simulink model "nonlinear_model"  (R2021a)
settings: Solver=ode2  StartTime=0.0  StopTime=40  FixedStep=0.001  RelTol=1e-3
values from neighbouring files (symbols this model uses):
  delta_elevator_max_down = 15 * (pi/180)    (= 0.261799387799)    [linear_and_nonlinear_model.m]    (also in linear_and_nonlinear_model_diff_speed_deff.m)
  delta_elevator_max_up = -21 * (pi/180)    (= -0.366519142919)    [linear_and_nonlinear_model.m]    (also in linear_and_nonlinear_model_diff_speed_deff.m)
  delta_elevator_rate_down = -24 * (pi/180)    (= -0.418879020479)    [linear_and_nonlinear_model.m]    (also in linear_and_nonlinear_model_diff_speed_deff.m = delta_elevator_rate_down_array(index_deff))
  delta_elevator_rate_up = 24 * (pi/180)    (= 0.418879020479)    [linear_and_nonlinear_model.m]    (also in linear_and_nonlinear_model_diff_speed_deff.m = delta_elevator_rate_up_array(index_deff))
  Delta_H_target = 100    [linear_and_nonlinear_model.m]    (also in linear_and_nonlinear_model_diff_speed_deff.m)
  i_H = 0.8*(1/(T_1c*V))    [epsilon_nu_find.m]    (also in short_period.m = 0.8*(1/(T_1c*V_target)))
  K_omega_z_int = get_K_value(K_omega_z_calc, q_calc, mach_calc_bode(i), H_calc_bode(i))    [short_period.m]
  K_theta_int = get_K_value(K_theta_calc, q_calc, mach_calc_bode(i), H_calc_bode(i))    [short_period.m]
  theta_max_down = -6.0 * (pi/180)    (= -0.10471975512)    [linear_and_nonlinear_model.m]    (also in linear_and_nonlinear_model_diff_speed_deff.m)
  theta_max_up = 6.0 * (pi/180)    (= 0.10471975512)    [linear_and_nonlinear_model.m]    (also in linear_and_nonlinear_model_diff_speed_deff.m)
libraries: cstblocks x5
settings Model: Creator=lalapopa  LastModifiedBy=lalapopa

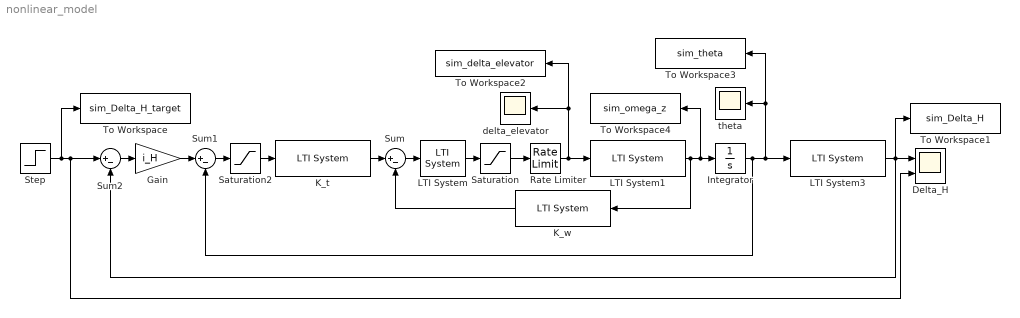
== system nonlinear_model ==
  Delta_H : Scope  NumInputPorts=2
  Gain : Gain  Gain=i_H
  Integrator : Integrator
  K_t : cstblocks/LTI System  sys=-K_theta_int  IC=[]
  K_w : cstblocks/LTI System  sys=-K_omega_z_int  IC=[]
  LTI System : cstblocks/LTI System  sys=W_p  IC=[]
  LTI System1 : cstblocks/LTI System  sys=d_w_d_v  IC=[]
  LTI System3 : cstblocks/LTI System  sys=W_H_theta  IC=[]
  Rate Limiter : RateLimiter  RisingSlewLimit=delta_elevator_rate_up  FallingSlewLimit=delta_elevator_rate_down  LinearizeAsGain=off
  Saturation : Saturate  UpperLimit=delta_elevator_max_down  LowerLimit=delta_elevator_max_up  LinearizeAsGain=off
  Saturation2 : Saturate  UpperLimit=theta_max_up  LowerLimit=theta_max_down  LinearizeAsGain=off
  Step : Step  After=Delta_H_target  SampleTime=0
  Sum : Sum  Inputs=|+-
  Sum1 : Sum  Inputs=|+-
  Sum2 : Sum  Inputs=|+-
  To Workspace : ToWorkspace  VariableName=sim_Delta_H_target  SaveFormat=Timeseries  SampleTime=-1
      settings: Decimation=3  Save2DSignal=2-D array (concatenate along first dimension)
  To Workspace1 : ToWorkspace  VariableName=sim_Delta_H  SaveFormat=Timeseries  SampleTime=-1
  To Workspace2 : ToWorkspace  VariableName=sim_delta_elevator  SaveFormat=Timeseries  SampleTime=-1
  To Workspace3 : ToWorkspace  VariableName=sim_theta  SaveFormat=Timeseries  SampleTime=-1
  To Workspace4 : ToWorkspace  VariableName=sim_omega_z  SaveFormat=Timeseries  SampleTime=-1
  delta_elevator : Scope
  theta : Scope
  wires:
  K_t/1 -> Sum/1
  Sum/1 -> LTI System/1
  K_w/1 -> Sum/2
  LTI System1/1 -> K_w/1, To Workspace4/1, Integrator/1
  LTI System3/1 -> Delta_H/1, Sum2/2, To Workspace1/1
  Integrator/1 -> To Workspace3/1, theta/1, LTI System3/1, Sum1/2
  LTI System/1 -> Saturation/1
  Saturation/1 -> Rate Limiter/1
  Rate Limiter/1 -> LTI System1/1, To Workspace2/1, delta_elevator/1
  Step/1 -> Delta_H/2, Sum2/1, To Workspace/1
  Sum2/1 -> Gain/1
  Sum1/1 -> Saturation2/1
  Saturation2/1 -> K_t/1
  Gain/1 -> Sum1/1
